simulink model "CCModel_61"  (R2024a)
settings: Solver=ode3  StartTime=0.0  StopTime=100  FixedStep=0.001  RelTol=1e-3  EnableMultiTasking=on
undefined symbols (not defined in the file or in its folder): DiscIntNeverNeededParam, Hecate_desVel1, Hecate_desVel2, Hecate_desVel3, Hecate_horShift, Hecate_period, Hecate_slope, Hecate_Transition1, Hecate_Transition2, Hecate_verShift, i, PME_qb, qb_map, RPM_qb, V
libraries: simulink x46
(part 4 of 11)

== system CCModel_61/Cruise Control/Version 5.0/Detect Change ==
  note: This subsystem detects either a change in the reference velocity, or the driver releasing one of the pedals. It outputs the time of the change, the value of u just before the change, and a boolean "hasChanged" value
  desired_velocity : Inport
  throttle_const : Inport  Port=2
  brake_const : Inport  Port=3
  Smoothed u : Inport  Port=4
  (False) : Constant  Value=0
  (True) : Constant
  AND : Logic  IconShape=distinctive  AllPortsSameDT=off  OutDataTypeStr=boolean
  Clock : Clock
  Delay : Delay  DelayLength=1
  Delay1 : Delay  DelayLength=1
  Detect Change : simulink/Logic and Bit Operations/Detect Change  vinit=0  OutDataTypeStr=boolean
  Detect Change1 : simulink/Logic and Bit Operations/Detect Change  vinit=0  OutDataTypeStr=boolean
  Max : MinMax  Function=max  Inputs=2
  OR : Logic  Operator=OR  IconShape=distinctive  AllPortsSameDT=off  OutDataTypeStr=boolean
  Pedal_threshold : Constant
  Scope : Scope
  Subtract : Sum  Inputs=+-
  Switch : Switch  Criteria=u2 > Threshold  SaturateOnIntegerOverflow=off  InputSameDT=off
  Switch1 : Switch  Criteria=u2 > Threshold  SaturateOnIntegerOverflow=off  InputSameDT=off
  Switch2 : Switch  Criteria=u2 > Threshold  SaturateOnIntegerOverflow=off  InputSameDT=off
  Change_time : Outport
  Old u : Outport  Port=2
  hasChanged : Outport  Port=3
  wires:
  desired_velocity/1 -> Detect Change/1
  Detect Change/1 -> OR/1
  OR/1 -> Switch/2, Switch2/2, hasChanged/1
  Switch1/1 -> Detect Change1/1, Delay1/1
  AND/1 -> OR/2
  Clock/1 -> Switch/1
  Max/1 -> Subtract/1
  (True)/1 -> Switch1/1
  brake_const/1 -> Max/2
  Pedal_threshold/1 -> Subtract/2
  Subtract/1 -> Switch1/2
  (False)/1 -> Switch1/3
  throttle_const/1 -> Max/1
  Switch2/1 -> Switch2/3, Old u/1
  Delay/1 -> Switch2/1
  Switch/1 -> Switch/3, Scope/1, Change_time/1
  Smoothed u/1 -> Delay/1
  Detect Change1/1 -> AND/2
  Delay1/1 -> AND/1

== system CCModel_61/Cruise Control/Version 5.0/PID Controller ==
  note: Typical PID controller, outputs a value between -100 and 100
  error : Inport
  Grade : Inport  Port=2
  Add : Sum
  Add1 : Sum
  Derivative : Derivative
  GKi : Gain  Gain=0
  GKp : Gain  Gain=3
  Integrator : Integrator
  Integrator1 : Integrator
  Kd : Gain  Gain=0.1
  Ki : Gain  Gain=0.03
  Kp : Gain  Gain=3
  Saturation : Saturate  UpperLimit=100  LowerLimit=-100
  Sum : Sum  Inputs=+++
  u : Outport
  wires:
  Integrator/1 -> Ki/1
  error/1 -> Integrator/1, Kp/1, Derivative/1  "D"
  Kp/1 -> Sum/2  "P"
  Ki/1 -> Sum/1  "I"
  Saturation/1 -> u/1
  Derivative/1 -> Kd/1
  Kd/1 -> Sum/3  "D"
  Sum/1 -> Add1/1
  Add1/1 -> Saturation/1
  Grade/1 -> Integrator1/1, GKp/1
  Integrator1/1 -> GKi/1
  GKi/1 -> Add/1
  GKp/1 -> Add/2
  Add/1 -> Add1/2

== system CCModel_61/Cruise Control/Version 5.0/Sigmoid ==
  note: This whole part is just to eliminate weird cancellation errors that were happening
  note: This system smooths out curves using the sigmoid equation shown above.
      | u1 is "Old u" which is the last value u had when change was detected.
      | u2 is "New u" which is the current output being given by the PID controller.
      | x is the time elapsed since the last change
      | k is the "sigmoid gain" which dictates how fast the transition occurs
  Change_time : Inport
  Old u : Inport  Port=2
  New u : Inport  Port=3
  Add : Sum
  Add1 : Sum
  Add2 : Sum
  Clock : Clock
  Constant : Constant
  Constant1 : Constant
  Constant2 : Constant
  Divide : Product  Inputs=/*
  Divide1 : Product  Inputs=**
  Divide2 : Product  Inputs=/*
  Divide3 : Product  Inputs=**
  Gain : Gain  Gain=1000
  Gain1 : Gain  Gain=0.001
  K : Constant  Value=1.5
  Power{,1..3} (4 alike) : Math  Operator=pow
  Reciprocal : Product  Inputs=/
  Reciprocal1 : Product  Inputs=/
  Round : Rounding  Operator=round
  Scope : Scope  NumInputPorts=3
  Subtract : Sum  Inputs=-+
  Sum : Sum  Inputs=|-+
  u_out : Outport
  wires:
  Power1/1 -> Scope/3, Add/1
  Add/1 -> Power/1
  Clock/1 -> Sum/2
  Constant/1 -> Add/2
  Sum/1 -> Gain/1  "Elapsed Time"
  Reciprocal/1 -> Power/2
  Power/1 -> Divide/1
  Divide/1 -> Divide1/1  "Sigmoid Function"
  Add1/1 -> Power2/1
  Power3/1 -> Add1/1
  K/1 -> Scope/2, Reciprocal/1, Power1/2, Reciprocal1/1, Power3/2
  Reciprocal1/1 -> Power2/2
  Power2/1 -> Divide2/1
  Constant1/1 -> Add1/2
  Change_time/1 -> Sum/1
  Constant2/1 -> Subtract/2
  Divide2/1 -> Subtract/1  "Sigmoid Function"
  Divide1/1 -> Add2/1
  Add2/1 -> u_out/1
  New u/1 -> Divide1/2
  Old u/1 -> Divide3/2
  Subtract/1 -> Divide3/1
  Divide3/1 -> Add2/2
  Gain1/1 -> Power1/1, Divide/2, Scope/1, Divide2/2, Power3/1
  Gain/1 -> Round/1
  Round/1 -> Gain1/1

== system CCModel_61/Cruise Control/Version 5.0/Switches ==
  note: This subsystem determines the source of input, either the cruise control or the driver
      | It also determines for a given u if the brake or throttle should be applied
      | Lastly, it smooths out the cruise control brakes and throttles to prevent jerk peaks
  note: Apply sigmoid curving to the throttle and brake
  note: If u is positive, throttle is applied
      | If u is negative, brake is applied
      | Max gains prevent large jerks from happening
  note: If throttle or brake are above 5 the driver takes control of the system
  throttle_const : Inport
  u : Inport  Port=2
  brake_const : Inport  Port=3
  hasChanged : Inport  Port=4
  Grade : Inport  Port=5
  (False) : Constant  Value=0
  (True) : Constant
  Brake_Switch : Switch  Criteria=u2 > Threshold  SaturateOnIntegerOverflow=off  InputSameDT=off
  Brake_Switch2 : Switch  Criteria=u2 > Threshold  SaturateOnIntegerOverflow=off  InputSameDT=off
  Clock : Clock
  Clock1 : Clock
  Constant : Constant
  Constant3 : Constant  Value=0
  Delay1 : Delay  DelayLength=1
  Delay3 : Delay  DelayLength=1
  Gain : Gain  Gain=1/150
  Gain1 : Gain  Gain=4
  Gain2 : Gain  Gain=-1
  Max : MinMax  Function=max  Inputs=2
  Max Brake : Gain  Gain=-0.5
  Max Throttle : Gain  Commented=through  Gain=0.8
  Pedal_threshold : Constant  Value=5
  Sigmoid_brake : Subsystem
  Sigmoid_throttle : Subsystem
  Sqrt : Sqrt
  Square : Math  Operator=square
  Subtract : Sum  Inputs=+-
  Switch : Switch  Criteria=u2 > Threshold  SaturateOnIntegerOverflow=off  InputSameDT=off
  Switch{1..4} (4 alike) : Switch  Criteria=u2 > Threshold  Threshold=0.04  SaturateOnIntegerOverflow=off  InputSameDT=off
  Switch5 : Switch  Criteria=u2 > Threshold  SaturateOnIntegerOverflow=off  InputSameDT=off
  Switch6 : Switch  Criteria=u2 > Threshold  Threshold=2.5  SaturateOnIntegerOverflow=off  InputSameDT=off
  Throttle_Switch : Switch  Criteria=u2 > Threshold  SaturateOnIntegerOverflow=off  InputSameDT=off
  Throttle_Switch2 : Switch  Criteria=u2 > Threshold  SaturateOnIntegerOverflow=off  InputSameDT=off
  Throttle : Outport
  Brake : Outport  Port=2
  Source : Outport  Port=3
  wires:
  throttle_const/1 -> Throttle_Switch2/1, Max/1
  brake_const/1 -> Max/2, Brake_Switch2/1
  Max/1 -> Subtract/1
  Pedal_threshold/1 -> Subtract/2
  Subtract/1 -> Switch/2
  (True)/1 -> Switch/1
  (False)/1 -> Switch/3
  Switch/1 -> Brake_Switch2/2, Throttle_Switch2/2, Source/1
  u/1 -> Throttle_Switch/2, Square/1, Brake_Switch/2, Max Brake/1, Gain2/1
  Constant3/1 -> Brake_Switch/1, Throttle_Switch/3
  Throttle_Switch2/1 -> Throttle/1
  Brake_Switch2/1 -> Brake/1
  Switch1/1 -> Switch1/3, Sigmoid_throttle/1(Change_time)  "Time"
  Switch2/1 -> Switch2/3, Sigmoid_throttle/2(Old thr)  "Old throttle"
  Throttle_Switch/1 -> Sigmoid_throttle/3(New thr)  "Throttle"
  Sigmoid_throttle/1(throttle_out) -> Delay1/1, Throttle_Switch2/3  "Smoothed throttle"
  Clock/1 -> Switch1/1
  hasChanged/1 -> Switch4/2, Switch3/2, Switch1/2, Switch2/2
  Delay1/1 -> Switch2/1
  Switch3/1 -> Switch3/3, Sigmoid_brake/1(Change_time)  "Time"
  Brake_Switch/1 -> Sigmoid_brake/3(New brake)  "Brake"
  Clock1/1 -> Switch3/1
  Switch4/1 -> Switch4/3, Sigmoid_brake/2(Old brake)  "Old brake"
  Delay3/1 -> Switch4/1
  Sigmoid_brake/1(brake_out) -> Delay3/1, Brake_Switch2/3  "Smoothed Brake"
  Square/1 -> Gain/1
  Sqrt/1 -> Gain1/1
  Gain2/1 -> Sqrt/1
  Gain/1 -> Throttle_Switch/1
  Grade/1 -> Switch5/2, Switch6/2
  Gain1/1 -> Switch5/3
  Max Brake/1 -> Switch6/3
  Switch6/1 -> Switch5/1
  Switch5/1 -> Brake_Switch/3
  Constant/1 -> Switch6/1

== system CCModel_61/Cruise Control/Version 6.0/Detect Change ==
  note: This subsystem detects either a change in the reference velocity, or the driver releasing one of the pedals. It outputs the time of the change, the value of u just before the change, and a boolean "hasChanged" value
  desired_velocity : Inport
  throttle_const : Inport  Port=2
  brake_const : Inport  Port=3
  Smoothed u : Inport  Port=4
  (False) : Constant  Value=0
  (True) : Constant
  AND : Logic  IconShape=distinctive  AllPortsSameDT=off  OutDataTypeStr=boolean
  Clock : Clock
  Delay : Delay  DelayLength=1
  Delay1 : Delay  DelayLength=1
  Detect Change : simulink/Logic and Bit Operations/Detect Change  vinit=0  OutDataTypeStr=boolean
  Detect Change1 : simulink/Logic and Bit Operations/Detect Change  vinit=0  OutDataTypeStr=boolean
  Max : MinMax  Function=max  Inputs=2
  OR : Logic  Operator=OR  IconShape=distinctive  AllPortsSameDT=off  OutDataTypeStr=boolean
  Pedal_threshold : Constant
  Scope : Scope
  Subtract : Sum  Inputs=+-
  Switch : Switch  Criteria=u2 > Threshold  SaturateOnIntegerOverflow=off  InputSameDT=off
  Switch1 : Switch  Criteria=u2 > Threshold  SaturateOnIntegerOverflow=off  InputSameDT=off
  Switch2 : Switch  Criteria=u2 > Threshold  SaturateOnIntegerOverflow=off  InputSameDT=off
  Change_time : Outport
  Old u : Outport  Port=2
  hasChanged : Outport  Port=3
  wires:
  desired_velocity/1 -> Detect Change/1
  Detect Change/1 -> OR/1
  OR/1 -> Switch/2, Switch2/2, hasChanged/1
  Switch1/1 -> Detect Change1/1, Delay1/1
  AND/1 -> OR/2
  Clock/1 -> Switch/1
  Max/1 -> Subtract/1
  (True)/1 -> Switch1/1
  brake_const/1 -> Max/2
  Pedal_threshold/1 -> Subtract/2
  Subtract/1 -> Switch1/2
  (False)/1 -> Switch1/3
  throttle_const/1 -> Max/1
  Switch2/1 -> Switch2/3, Old u/1
  Delay/1 -> Switch2/1
  Switch/1 -> Switch/3, Scope/1, Change_time/1
  Smoothed u/1 -> Delay/1
  Detect Change1/1 -> AND/2
  Delay1/1 -> AND/1

== system CCModel_61/Cruise Control/Version 6.0/PID Controller ==
  note: Typical PID controller, outputs a value between -100 and 100
  error : Inport
  Grade : Inport  Port=2
  Add : Sum
  Add1 : Sum
  Derivative : Derivative
  GKi : Gain  Gain=0
  GKp : Gain  Gain=0
  Integrator : Integrator
  Integrator1 : Integrator
  Kd : Gain  Gain=0.1
  Ki : Gain  Gain=0.03
  Kp : Gain  Gain=5
  Saturation : Saturate  UpperLimit=100  LowerLimit=-100
  Sum : Sum  Inputs=+++
  u : Outport
  wires:
  Integrator/1 -> Ki/1
  error/1 -> Integrator/1, Kp/1, Derivative/1  "D"
  Kp/1 -> Sum/2  "P"
  Ki/1 -> Sum/1  "I"
  Saturation/1 -> u/1
  Derivative/1 -> Kd/1
  Kd/1 -> Sum/3  "D"
  Sum/1 -> Add1/1
  Add1/1 -> Saturation/1
  Grade/1 -> Integrator1/1, GKp/1
  Integrator1/1 -> GKi/1
  GKi/1 -> Add/1
  GKp/1 -> Add/2
  Add/1 -> Add1/2

== system CCModel_61/Cruise Control/Version 6.0/Sigmoid ==
  note: This whole part is just to eliminate weird cancellation errors that were happening
  note: This system smooths out curves using the sigmoid equation shown above.
      | u1 is "Old u" which is the last value u had when change was detected.
      | u2 is "New u" which is the current output being given by the PID controller.
      | x is the time elapsed since the last change
      | k is the "sigmoid gain" which dictates how fast the transition occurs
  Change_time : Inport
  Old u : Inport  Port=2
  New u : Inport  Port=3
  Add : Sum
  Add1 : Sum
  Add2 : Sum
  Clock : Clock
  Constant : Constant
  Constant1 : Constant
  Constant2 : Constant
  Divide : Product  Inputs=/*
  Divide1 : Product  Inputs=**
  Divide2 : Product  Inputs=/*
  Divide3 : Product  Inputs=**
  Gain : Gain  Gain=1000
  Gain1 : Gain  Gain=0.001
  K : Constant  Value=1.5
  Power{,1..3} (4 alike) : Math  Operator=pow
  Reciprocal : Product  Inputs=/
  Reciprocal1 : Product  Inputs=/
  Round : Rounding  Operator=round
  Scope : Scope  NumInputPorts=3
  Subtract : Sum  Inputs=-+
  Sum : Sum  Inputs=|-+
  u_out : Outport
  wires:
  Power1/1 -> Scope/3, Add/1
  Add/1 -> Power/1
  Clock/1 -> Sum/2
  Constant/1 -> Add/2
  Sum/1 -> Gain/1  "Elapsed Time"
  Reciprocal/1 -> Power/2
  Power/1 -> Divide/1
  Divide/1 -> Divide1/1  "Sigmoid Function"
  Add1/1 -> Power2/1
  Power3/1 -> Add1/1
  K/1 -> Scope/2, Reciprocal/1, Power1/2, Reciprocal1/1, Power3/2
  Reciprocal1/1 -> Power2/2
  Power2/1 -> Divide2/1
  Constant1/1 -> Add1/2
  Change_time/1 -> Sum/1
  Constant2/1 -> Subtract/2
  Divide2/1 -> Subtract/1  "Sigmoid Function"
  Divide1/1 -> Add2/1
  Add2/1 -> u_out/1
  New u/1 -> Divide1/2
  Old u/1 -> Divide3/2
  Subtract/1 -> Divide3/1
  Divide3/1 -> Add2/2
  Gain1/1 -> Power1/1, Divide/2, Scope/1, Divide2/2, Power3/1
  Gain/1 -> Round/1
  Round/1 -> Gain1/1

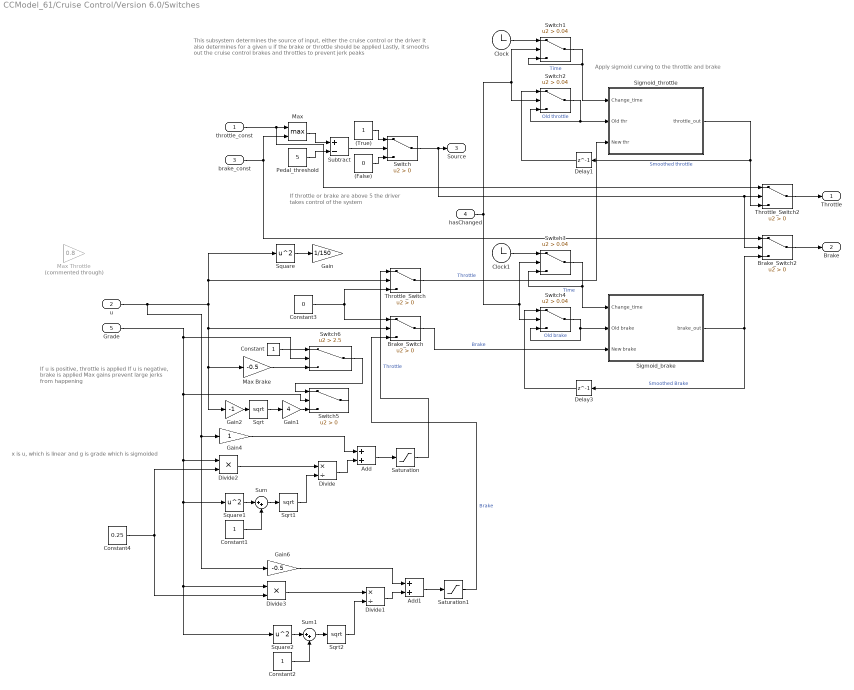
== system CCModel_61/Cruise Control/Version 6.0/Switches ==
  note: x is u, which is linear and g is grade which is sigmoided
  note: This subsystem determines the source of input, either the cruise control or the driver
      | It also determines for a given u if the brake or throttle should be applied
      | Lastly, it smooths out the cruise control brakes and throttles to prevent jerk peaks
  note: Apply sigmoid curving to the throttle and brake
  note: If u is positive, throttle is applied
      | If u is negative, brake is applied
      | Max gains prevent large jerks from happening
  note: If throttle or brake are above 5 the driver takes control of the system
  throttle_const : Inport
  u : Inport  Port=2
  brake_const : Inport  Port=3
  hasChanged : Inport  Port=4
  Grade : Inport  Port=5
  (False) : Constant  Value=0
  (True) : Constant
  Add : Sum
  Add1 : Sum
  Brake_Switch : Switch  Criteria=u2 > Threshold  SaturateOnIntegerOverflow=off  InputSameDT=off
  Brake_Switch2 : Switch  Criteria=u2 > Threshold  SaturateOnIntegerOverflow=off  InputSameDT=off
  Clock : Clock
  Clock1 : Clock
  Constant : Constant
  Constant1 : Constant
  Constant2 : Constant
  Constant3 : Constant  Value=0
  Constant4 : Constant  Value=0.25
  Delay1 : Delay  DelayLength=1
  Delay3 : Delay  DelayLength=1
  Divide : Product  Inputs=*/
  Divide1 : Product  Inputs=*/
  Divide2 : Product  Inputs=**
  Divide3 : Product  Inputs=**
  Gain : Gain  Gain=1/150
  Gain1 : Gain  Gain=4
  Gain2 : Gain  Gain=-1
  Gain4 : Gain
  Gain6 : Gain  Gain=-0.5
  Max : MinMax  Function=max  Inputs=2
  Max Brake : Gain  Gain=-0.5
  Max Throttle : Gain  Commented=through  Gain=0.8
  Pedal_threshold : Constant  Value=5
  Saturation : Saturate  UpperLimit=100  LowerLimit=0
  Saturation1 : Saturate  UpperLimit=100  LowerLimit=0
  Sigmoid_brake : Subsystem
  Sigmoid_throttle : Subsystem
  Sqrt : Sqrt
  Sqrt1 : Sqrt
  Sqrt2 : Sqrt
  Square : Math  Operator=square
  Square1 : Math  Operator=square
  Square2 : Math  Operator=square
  Subtract : Sum  Inputs=+-
  Sum : Sum  Inputs=|++
  Sum1 : Sum  Inputs=|++
  Switch : Switch  Criteria=u2 > Threshold  SaturateOnIntegerOverflow=off  InputSameDT=off
  Switch{1..4} (4 alike) : Switch  Criteria=u2 > Threshold  Threshold=0.04  SaturateOnIntegerOverflow=off  InputSameDT=off
  Switch5 : Switch  Criteria=u2 > Threshold  SaturateOnIntegerOverflow=off  InputSameDT=off
  Switch6 : Switch  Criteria=u2 > Threshold  Threshold=2.5  SaturateOnIntegerOverflow=off  InputSameDT=off
  Throttle_Switch : Switch  Criteria=u2 > Threshold  SaturateOnIntegerOverflow=off  InputSameDT=off
  Throttle_Switch2 : Switch  Criteria=u2 > Threshold  SaturateOnIntegerOverflow=off  InputSameDT=off
  Throttle : Outport
  Brake : Outport  Port=2
  Source : Outport  Port=3
  wires:
  throttle_const/1 -> Throttle_Switch2/1, Max/1
  brake_const/1 -> Max/2, Brake_Switch2/1
  Max/1 -> Subtract/1
  Pedal_threshold/1 -> Subtract/2
  Subtract/1 -> Switch/2
  (True)/1 -> Switch/1
  (False)/1 -> Switch/3
  Switch/1 -> Brake_Switch2/2, Throttle_Switch2/2, Source/1
  u/1 -> Gain6/1, Gain4/1, Throttle_Switch/2, Square/1, Brake_Switch/2, Max Brake/1, Gain2/1
  Constant3/1 -> Brake_Switch/1, Throttle_Switch/3
  Throttle_Switch2/1 -> Throttle/1
  Brake_Switch2/1 -> Brake/1
  Switch1/1 -> Switch1/3, Sigmoid_throttle/1(Change_time)  "Time"
  Switch2/1 -> Switch2/3, Sigmoid_throttle/2(Old thr)  "Old throttle"
  Throttle_Switch/1 -> Sigmoid_throttle/3(New thr)  "Throttle"
  Sigmoid_throttle/1(throttle_out) -> Delay1/1, Throttle_Switch2/3  "Smoothed throttle"
  Clock/1 -> Switch1/1
  hasChanged/1 -> Switch4/2, Switch3/2, Switch1/2, Switch2/2
  Delay1/1 -> Switch2/1
  Switch3/1 -> Switch3/3, Sigmoid_brake/1(Change_time)  "Time"
  Brake_Switch/1 -> Sigmoid_brake/3(New brake)  "Brake"
  Clock1/1 -> Switch3/1
  Switch4/1 -> Switch4/3, Sigmoid_brake/2(Old brake)  "Old brake"
  Delay3/1 -> Switch4/1
  Sigmoid_brake/1(brake_out) -> Delay3/1, Brake_Switch2/3  "Smoothed Brake"
  Square/1 -> Gain/1
  Sqrt/1 -> Gain1/1
  Gain2/1 -> Sqrt/1
  Gain1/1 -> Switch5/3
  Max Brake/1 -> Switch6/3
  Switch6/1 -> Switch5/1
  Constant/1 -> Switch6/1
  Square1/1 -> Sum/1
  Constant1/1 -> Sum/2
  Sum/1 -> Sqrt1/1
  Divide2/1 -> Divide/1
  Sqrt1/1 -> Divide/2
  Gain4/1 -> Add/1
  Divide/1 -> Add/2
  Add/1 -> Saturation/1
  Saturation/1 -> Throttle_Switch/1  "Throttle"
  Square2/1 -> Sum1/1
  Gain6/1 -> Add1/1
  Divide1/1 -> Add1/2
  Constant2/1 -> Sum1/2
  Divide3/1 -> Divide1/1
  Sum1/1 -> Sqrt2/1
  Add1/1 -> Saturation1/1
  Sqrt2/1 -> Divide1/2
  Grade/1 -> Switch5/2, Divide2/1, Square1/1, Divide3/1, Square2/1, Switch6/2
  Saturation1/1 -> Brake_Switch/3  "Brake"
  Constant4/1 -> Divide3/2, Divide2/2

== system CCModel_61/Cruise Control/Version 6.1/Detect Change ==
  note: This subsystem detects either a change in the reference velocity, or the driver releasing one of the pedals. It outputs the time of the change, the value of u just before the change, and a boolean "hasChanged" value
  desired_velocity : Inport
  throttle_const : Inport  Port=2
  brake_const : Inport  Port=3
  Smoothed u : Inport  Port=4
  (False) : Constant  Value=0
  (True) : Constant
  AND : Logic  IconShape=distinctive  AllPortsSameDT=off  OutDataTypeStr=boolean
  Clock : Clock
  Delay : Delay  DelayLength=1
  Delay1 : Delay  DelayLength=1
  Detect Change : simulink/Logic and Bit Operations/Detect Change  vinit=0  OutDataTypeStr=boolean
  Detect Change1 : simulink/Logic and Bit Operations/Detect Change  vinit=0  OutDataTypeStr=boolean
  Max : MinMax  Function=max  Inputs=2
  OR : Logic  Operator=OR  IconShape=distinctive  AllPortsSameDT=off  OutDataTypeStr=boolean
  Pedal_threshold : Constant
  Scope : Scope
  Subtract : Sum  Inputs=+-
  Switch : Switch  Criteria=u2 > Threshold  SaturateOnIntegerOverflow=off  InputSameDT=off
  Switch1 : Switch  Criteria=u2 > Threshold  SaturateOnIntegerOverflow=off  InputSameDT=off
  Switch2 : Switch  Criteria=u2 > Threshold  SaturateOnIntegerOverflow=off  InputSameDT=off
  Change_time : Outport
  Old u : Outport  Port=2
  hasChanged : Outport  Port=3
  wires:
  desired_velocity/1 -> Detect Change/1
  Detect Change/1 -> OR/1
  OR/1 -> Switch/2, Switch2/2, hasChanged/1
  Switch1/1 -> Detect Change1/1, Delay1/1
  AND/1 -> OR/2
  Clock/1 -> Switch/1
  Max/1 -> Subtract/1
  (True)/1 -> Switch1/1
  brake_const/1 -> Max/2
  Pedal_threshold/1 -> Subtract/2
  Subtract/1 -> Switch1/2
  (False)/1 -> Switch1/3
  throttle_const/1 -> Max/1
  Switch2/1 -> Switch2/3, Old u/1
  Delay/1 -> Switch2/1
  Switch/1 -> Switch/3, Scope/1, Change_time/1
  Smoothed u/1 -> Delay/1
  Detect Change1/1 -> AND/2
  Delay1/1 -> AND/1

== system CCModel_61/Cruise Control/Version 6.1/PID Controller ==
  note: Typical PID controller, outputs a value between -100 and 100
  error : Inport
  Grade : Inport  Port=2
  Add : Sum
  Add1 : Sum
  Derivative : Derivative
  GKi : Gain  Gain=0
  GKp : Gain  Gain=0
  Integrator : Integrator
  Integrator1 : Integrator
  Kd : Gain  Gain=0.1
  Ki : Gain  Gain=0.03
  Kp : Gain  Gain=3
  Saturation : Saturate  UpperLimit=100  LowerLimit=-100
  Scope : Scope  NumInputPorts=2
  Scope1 : Scope  NumInputPorts=3
  Sum : Sum  Inputs=+++
  u : Outport
  P : Outport  Port=2
  wires:
  Integrator/1 -> Ki/1
  error/1 -> Scope/1, Integrator/1, Kp/1, Derivative/1  "D"
  Kp/1 -> P/1, Scope1/1, Sum/2  "P"
  Ki/1 -> Sum/1, Scope1/2  "I"
  Saturation/1 -> u/1
  Derivative/1 -> Kd/1
  Kd/1 -> Scope1/3, Sum/3  "D"
  Sum/1 -> Add1/1, Scope/2
  Add1/1 -> Saturation/1
  Grade/1 -> Integrator1/1, GKp/1
  Integrator1/1 -> GKi/1
  GKi/1 -> Add/1
  GKp/1 -> Add/2
  Add/1 -> Add1/2

== system CCModel_61/Cruise Control/Version 6.1/Sigmoid ==
  note: This whole part is just to eliminate weird cancellation errors that were happening
  note: This system smooths out curves using the sigmoid equation shown above.
      | u1 is "Old u" which is the last value u had when change was detected.
      | u2 is "New u" which is the current output being given by the PID controller.
      | x is the time elapsed since the last change
      | k is the "sigmoid gain" which dictates how fast the transition occurs
  Change_time : Inport
  Old u : Inport  Port=2
  New u : Inport  Port=3
  Add : Sum
  Add1 : Sum
  Add2 : Sum
  Clock : Clock
  Constant : Constant
  Constant1 : Constant
  Constant2 : Constant
  Divide : Product  Inputs=/*
  Divide1 : Product  Inputs=**
  Divide2 : Product  Inputs=/*
  Divide3 : Product  Inputs=**
  Gain : Gain  Gain=1000
  Gain1 : Gain  Gain=0.001
  K : Constant  Value=1.5
  Power{,1..3} (4 alike) : Math  Operator=pow
  Reciprocal : Product  Inputs=/
  Reciprocal1 : Product  Inputs=/
  Round : Rounding  Operator=round
  Scope : Scope  NumInputPorts=3
  Subtract : Sum  Inputs=-+
  Sum : Sum  Inputs=|-+
  u_out : Outport
  wires:
  Power1/1 -> Scope/3, Add/1
  Add/1 -> Power/1
  Clock/1 -> Sum/2
  Constant/1 -> Add/2
  Sum/1 -> Gain/1  "Elapsed Time"
  Reciprocal/1 -> Power/2
  Power/1 -> Divide/1
  Divide/1 -> Divide1/1  "Sigmoid Function"
  Add1/1 -> Power2/1
  Power3/1 -> Add1/1
  K/1 -> Scope/2, Reciprocal/1, Power1/2, Reciprocal1/1, Power3/2
  Reciprocal1/1 -> Power2/2
  Power2/1 -> Divide2/1
  Constant1/1 -> Add1/2
  Change_time/1 -> Sum/1
  Constant2/1 -> Subtract/2
  Divide2/1 -> Subtract/1  "Sigmoid Function"
  Divide1/1 -> Add2/1
  Add2/1 -> u_out/1
  New u/1 -> Divide1/2
  Old u/1 -> Divide3/2
  Subtract/1 -> Divide3/1
  Divide3/1 -> Add2/2
  Gain1/1 -> Power1/1, Divide/2, Scope/1, Divide2/2, Power3/1
  Gain/1 -> Round/1
  Round/1 -> Gain1/1

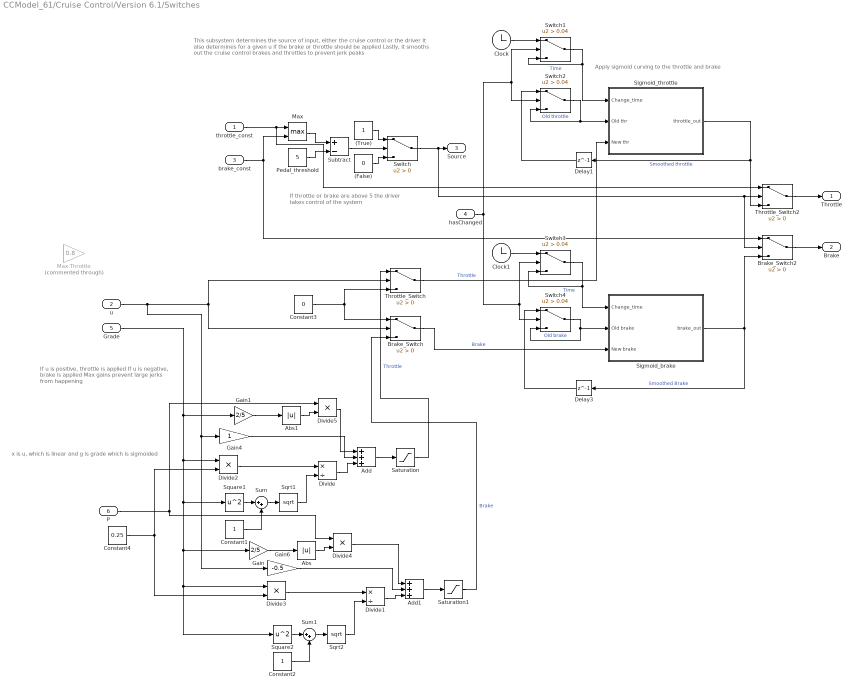
== system CCModel_61/Cruise Control/Version 6.1/Switches ==
  note: x is u, which is linear and g is grade which is sigmoided
  note: This subsystem determines the source of input, either the cruise control or the driver
      | It also determines for a given u if the brake or throttle should be applied
      | Lastly, it smooths out the cruise control brakes and throttles to prevent jerk peaks
  note: Apply sigmoid curving to the throttle and brake
  note: If u is positive, throttle is applied
      | If u is negative, brake is applied
      | Max gains prevent large jerks from happening
  note: If throttle or brake are above 5 the driver takes control of the system
  throttle_const : Inport
  u : Inport  Port=2
  brake_const : Inport  Port=3
  hasChanged : Inport  Port=4
  Grade : Inport  Port=5
  P : Inport  Port=6
  (False) : Constant  Value=0
  (True) : Constant
  Abs : Abs  SaturateOnIntegerOverflow=off
  Abs1 : Abs  SaturateOnIntegerOverflow=off
  Add : Sum  Inputs=+++
  Add1 : Sum  Inputs=+++
  Brake_Switch : Switch  Criteria=u2 > Threshold  SaturateOnIntegerOverflow=off  InputSameDT=off
  Brake_Switch2 : Switch  Criteria=u2 > Threshold  SaturateOnIntegerOverflow=off  InputSameDT=off
  Clock : Clock
  Clock1 : Clock
  Constant1 : Constant
  Constant2 : Constant
  Constant3 : Constant  Value=0
  Constant4 : Constant  Value=0.25
  Delay1 : Delay  DelayLength=1
  Delay3 : Delay  DelayLength=1
  Divide : Product  Inputs=*/
  Divide1 : Product  Inputs=*/
  Divide{2..5} (4 alike) : Product  Inputs=**
  Gain : Gain  Gain=2/5
  Gain1 : Gain  Gain=2/5
  Gain4 : Gain
  Gain6 : Gain  Gain=-0.5
  Max : MinMax  Function=max  Inputs=2
  Max Throttle : Gain  Commented=through  Gain=0.8
  Pedal_threshold : Constant  Value=5
  Saturation : Saturate  UpperLimit=100  LowerLimit=0
  Saturation1 : Saturate  UpperLimit=100  LowerLimit=0
  Sigmoid_brake : Subsystem
  Sigmoid_throttle : Subsystem
  Sqrt1 : Sqrt
  Sqrt2 : Sqrt
  Square1 : Math  Operator=square
  Square2 : Math  Operator=square
  Subtract : Sum  Inputs=+-
  Sum : Sum  Inputs=|++
  Sum1 : Sum  Inputs=|++
  Switch : Switch  Criteria=u2 > Threshold  SaturateOnIntegerOverflow=off  InputSameDT=off
  Switch{1..4} (4 alike) : Switch  Criteria=u2 > Threshold  Threshold=0.04  SaturateOnIntegerOverflow=off  InputSameDT=off
  Throttle_Switch : Switch  Criteria=u2 > Threshold  SaturateOnIntegerOverflow=off  InputSameDT=off
  Throttle_Switch2 : Switch  Criteria=u2 > Threshold  SaturateOnIntegerOverflow=off  InputSameDT=off
  Throttle : Outport
  Brake : Outport  Port=2
  Source : Outport  Port=3
  wires:
  throttle_const/1 -> Throttle_Switch2/1, Max/1
  brake_const/1 -> Max/2, Brake_Switch2/1
  Max/1 -> Subtract/1
  Pedal_threshold/1 -> Subtract/2
  Subtract/1 -> Switch/2
  (True)/1 -> Switch/1
  (False)/1 -> Switch/3
  Switch/1 -> Brake_Switch2/2, Throttle_Switch2/2, Source/1
  u/1 -> Gain6/1, Gain4/1, Throttle_Switch/2, Brake_Switch/2
  Constant3/1 -> Brake_Switch/1, Throttle_Switch/3
  Throttle_Switch2/1 -> Throttle/1
  Brake_Switch2/1 -> Brake/1
  Switch1/1 -> Switch1/3, Sigmoid_throttle/1(Change_time)  "Time"
  Switch2/1 -> Switch2/3, Sigmoid_throttle/2(Old thr)  "Old throttle"
  Throttle_Switch/1 -> Sigmoid_throttle/3(New thr)  "Throttle"
  Sigmoid_throttle/1(throttle_out) -> Delay1/1, Throttle_Switch2/3  "Smoothed throttle"
  Clock/1 -> Switch1/1
  hasChanged/1 -> Switch4/2, Switch3/2, Switch1/2, Switch2/2
  Delay1/1 -> Switch2/1
  Switch3/1 -> Switch3/3, Sigmoid_brake/1(Change_time)  "Time"
  Brake_Switch/1 -> Sigmoid_brake/3(New brake)  "Brake"
  Clock1/1 -> Switch3/1
  Switch4/1 -> Switch4/3, Sigmoid_brake/2(Old brake)  "Old brake"
  Delay3/1 -> Switch4/1
  Sigmoid_brake/1(brake_out) -> Delay3/1, Brake_Switch2/3  "Smoothed Brake"
  Square1/1 -> Sum/1
  Constant1/1 -> Sum/2
  Sum/1 -> Sqrt1/1
  Divide2/1 -> Divide/1
  Sqrt1/1 -> Divide/2
  Gain4/1 -> Add/2
  Divide/1 -> Add/3
  Add/1 -> Saturation/1
  Saturation/1 -> Throttle_Switch/1  "Throttle"
  Square2/1 -> Sum1/1
  Gain6/1 -> Add1/2
  Divide1/1 -> Add1/3
  Constant2/1 -> Sum1/2
  Divide3/1 -> Divide1/1
  Sum1/1 -> Sqrt2/1
  Add1/1 -> Saturation1/1
  Sqrt2/1 -> Divide1/2
  Grade/1 -> Gain1/1, Divide2/1, Square1/1, Gain/1, Divide3/1, Square2/1
  Saturation1/1 -> Brake_Switch/3  "Brake"
  Constant4/1 -> Divide3/2, Divide2/2
  Divide4/1 -> Add1/1
  Gain/1 -> Abs/1
  Abs/1 -> Divide4/2
  Abs1/1 -> Divide5/2
  Gain1/1 -> Abs1/1
  Divide5/1 -> Add/1
  P/1 -> Divide4/1, Divide5/1

== system CCModel_61/Cruise Control/Version 6.2/Detect Change ==
  note: This subsystem detects either a change in the reference velocity, or the driver releasing one of the pedals. It outputs the time of the change, the value of u just before the change, and a boolean "hasChanged" value
  desired_velocity : Inport
  throttle_const : Inport  Port=2
  brake_const : Inport  Port=3
  Smoothed u : Inport  Port=4
  (False) : Constant  Value=0
  (True) : Constant
  AND : Logic  IconShape=distinctive  AllPortsSameDT=off  OutDataTypeStr=boolean
  Clock : Clock
  Delay{,1..3} (4 alike) : Delay  DelayLength=1
  Detect Change : simulink/Logic and Bit Operations/Detect Change  vinit=0  OutDataTypeStr=boolean
  Detect Change1 : simulink/Logic and Bit Operations/Detect Change  vinit=0  OutDataTypeStr=boolean
  Max : MinMax  Function=max  Inputs=2
  OR : Logic  Operator=OR  IconShape=distinctive  AllPortsSameDT=off  OutDataTypeStr=boolean
  Pedal_threshold : Constant
  Scope : Scope
  Subtract : Sum  Inputs=+-
  Switch : Switch  Criteria=u2 > Threshold  SaturateOnIntegerOverflow=off  InputSameDT=off
  Switch1 : Switch  Criteria=u2 > Threshold  SaturateOnIntegerOverflow=off  InputSameDT=off
  Switch2 : Switch  Criteria=u2 > Threshold  SaturateOnIntegerOverflow=off  InputSameDT=off
  Change_time : Outport
  Old u : Outport  Port=2
  hasChanged : Outport  Port=3
  wires:
  desired_velocity/1 -> Detect Change/1
  Detect Change/1 -> OR/1
  OR/1 -> Switch/2, Switch2/2, hasChanged/1
  Switch1/1 -> Detect Change1/1, Delay1/1
  AND/1 -> OR/2
  Clock/1 -> Switch/1
  Max/1 -> Subtract/1
  (True)/1 -> Switch1/1
  brake_const/1 -> Max/2
  Pedal_threshold/1 -> Subtract/2
  Subtract/1 -> Switch1/2
  (False)/1 -> Switch1/3
  throttle_const/1 -> Max/1
  Switch2/1 -> Delay3/1, Old u/1
  Delay/1 -> Switch2/1
  Switch/1 -> Delay2/1, Scope/1, Change_time/1
  Smoothed u/1 -> Delay/1
  Detect Change1/1 -> AND/2
  Delay1/1 -> AND/1
  Delay2/1 -> Switch/3
  Delay3/1 -> Switch2/3

== system CCModel_61/Cruise Control/Version 6.2/PID Controller ==
  note: Typical PID controller, outputs a value between -100 and 100
  error : Inport
  Grade : Inport  Port=2
  Add : Sum
  Add1 : Sum
  Derivative : Derivative
  GKi : Gain  Gain=0
  GKp : Gain  Gain=0
  Integrator : Integrator
  Integrator1 : Integrator
  Kd : Gain  Gain=0.1
  Ki : Gain  Gain=0.03
  Kp : Gain  Gain=3
  Saturation : Saturate  UpperLimit=100  LowerLimit=-100
  Scope : Scope  NumInputPorts=2
  Scope1 : Scope  NumInputPorts=3
  Sum : Sum  Inputs=+++
  u : Outport
  P : Outport  Port=2
  wires:
  Integrator/1 -> Ki/1
  error/1 -> Scope/1, Integrator/1, Kp/1, Derivative/1  "D"
  Kp/1 -> P/1, Scope1/1, Sum/2  "P"
  Ki/1 -> Sum/1, Scope1/2  "I"
  Saturation/1 -> u/1
  Derivative/1 -> Kd/1
  Kd/1 -> Scope1/3, Sum/3  "D"
  Sum/1 -> Add1/1, Scope/2
  Add1/1 -> Saturation/1
  Grade/1 -> Integrator1/1, GKp/1
  Integrator1/1 -> GKi/1
  GKi/1 -> Add/1
  GKp/1 -> Add/2
  Add/1 -> Add1/2

== system CCModel_61/Cruise Control/Version 6.2/Sigmoid ==
  note: This whole part is just to eliminate weird cancellation errors that were happening
  note: This system smooths out curves using the sigmoid equation shown above.
      | u1 is "Old u" which is the last value u had when change was detected.
      | u2 is "New u" which is the current output being given by the PID controller.
      | x is the time elapsed since the last change
      | k is the "sigmoid gain" which dictates how fast the transition occurs
  Change_time : Inport
  Old u : Inport  Port=2
  New u : Inport  Port=3
  Add : Sum
  Add1 : Sum
  Add2 : Sum
  Clock : Clock
  Constant : Constant
  Constant1 : Constant
  Constant2 : Constant
  Divide : Product  Inputs=/*
  Divide1 : Product  Inputs=**
  Divide2 : Product  Inputs=/*
  Divide3 : Product  Inputs=**
  Gain : Gain  Gain=1000
  Gain1 : Gain  Gain=0.001
  K : Constant  Value=1.5
  Power{,1..3} (4 alike) : Math  Operator=pow
  Reciprocal : Product  Inputs=/
  Reciprocal1 : Product  Inputs=/
  Round : Rounding  Operator=round
  Scope : Scope  NumInputPorts=3
  Subtract : Sum  Inputs=-+
  Sum : Sum  Inputs=|-+
  u_out : Outport
  wires:
  Power1/1 -> Scope/3, Add/1
  Add/1 -> Power/1
  Clock/1 -> Sum/2
  Constant/1 -> Add/2
  Sum/1 -> Gain/1  "Elapsed Time"
  Reciprocal/1 -> Power/2
  Power/1 -> Divide/1
  Divide/1 -> Divide1/1  "Sigmoid Function"
  Add1/1 -> Power2/1
  Power3/1 -> Add1/1
  K/1 -> Scope/2, Reciprocal/1, Power1/2, Reciprocal1/1, Power3/2
  Reciprocal1/1 -> Power2/2
  Power2/1 -> Divide2/1
  Constant1/1 -> Add1/2
  Change_time/1 -> Sum/1
  Constant2/1 -> Subtract/2
  Divide2/1 -> Subtract/1  "Sigmoid Function"
  Divide1/1 -> Add2/1
  Add2/1 -> u_out/1
  New u/1 -> Divide1/2
  Old u/1 -> Divide3/2
  Subtract/1 -> Divide3/1
  Divide3/1 -> Add2/2
  Gain1/1 -> Power1/1, Divide/2, Scope/1, Divide2/2, Power3/1
  Gain/1 -> Round/1
  Round/1 -> Gain1/1

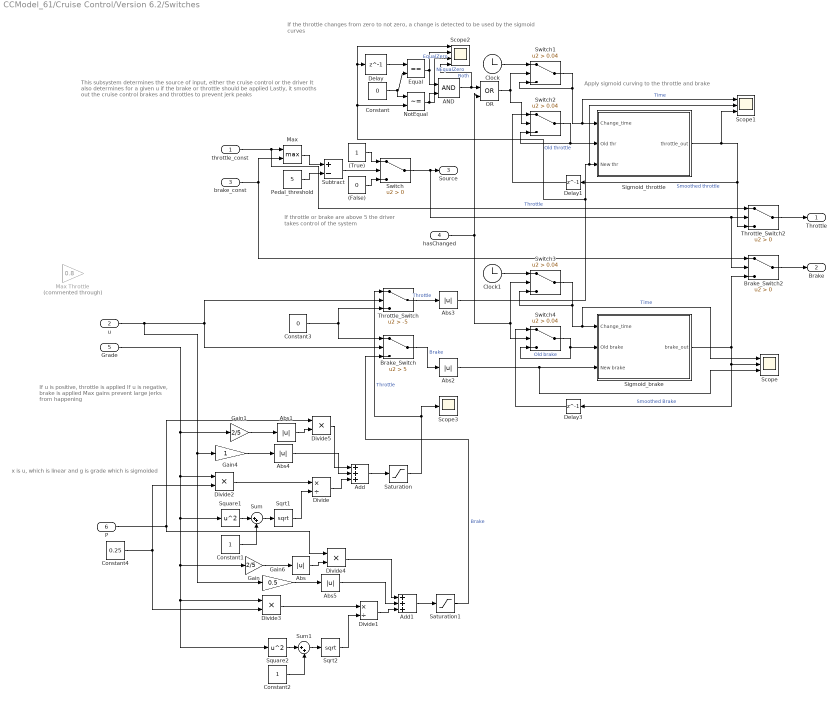
== system CCModel_61/Cruise Control/Version 6.2/Switches ==
  note: If the throttle changes from zero to not zero, a change is detected to be used by the sigmoid curves
  note: x is u, which is linear and g is grade which is sigmoided
  note: This subsystem determines the source of input, either the cruise control or the driver
      | It also determines for a given u if the brake or throttle should be applied
      | Lastly, it smooths out the cruise control brakes and throttles to prevent jerk peaks
  note: Apply sigmoid curving to the throttle and brake
  note: If u is positive, throttle is applied
      | If u is negative, brake is applied
      | Max gains prevent large jerks from happening
  note: If throttle or brake are above 5 the driver takes control of the system
  throttle_const : Inport
  u : Inport  Port=2
  brake_const : Inport  Port=3
  hasChanged : Inport  Port=4
  Grade : Inport  Port=5
  P : Inport  Port=6
  (False) : Constant  Value=0
  (True) : Constant
  AND : Logic  IconShape=distinctive  AllPortsSameDT=off  OutDataTypeStr=boolean
  Abs{,1..5} (6 alike) : Abs  SaturateOnIntegerOverflow=off
  Add : Sum  Inputs=+++
  Add1 : Sum  Inputs=+++
  Brake_Switch : Switch  Criteria=u2 > Threshold  Threshold=5  SaturateOnIntegerOverflow=off  InputSameDT=off
  Brake_Switch2 : Switch  Criteria=u2 > Threshold  SaturateOnIntegerOverflow=off  InputSameDT=off
  Clock : Clock
  Clock1 : Clock
  Constant : Constant  Value=0
  Constant1 : Constant
  Constant2 : Constant
  Constant3 : Constant  Value=0
  Constant4 : Constant  Value=0.25
  Delay : Delay  DelayLength=1
  Delay1 : Delay  DelayLength=1
  Delay3 : Delay  DelayLength=1
  Divide : Product  Inputs=*/
  Divide1 : Product  Inputs=*/
  Divide{2..5} (4 alike) : Product  Inputs=**
  Equal : RelationalOperator  Operator===  OutDataTypeStr=boolean  RndMeth=Simplest  InputSameDT=off
  Gain : Gain  Gain=2/5
  Gain1 : Gain  Gain=2/5
  Gain4 : Gain
  Gain6 : Gain  Gain=0.5
  Max : MinMax  Function=max  Inputs=2
  Max Throttle : Gain  Commented=through  Gain=0.8
  NotEqual : RelationalOperator  Operator=~=  OutDataTypeStr=boolean  RndMeth=Simplest  InputSameDT=off
  OR : Logic  Operator=OR  IconShape=distinctive  AllPortsSameDT=off  OutDataTypeStr=boolean
  Pedal_threshold : Constant  Value=5
  Saturation : Saturate  UpperLimit=100  LowerLimit=0
  Saturation1 : Saturate  UpperLimit=100  LowerLimit=0
  Scope : Scope  NumInputPorts=3
  Scope1 : Scope  NumInputPorts=3
  Scope2 : Scope  NumInputPorts=4
  Scope3 : Scope
  Sigmoid_brake : Subsystem
  Sigmoid_throttle : Subsystem
  Sqrt1 : Sqrt
  Sqrt2 : Sqrt
  Square1 : Math  Operator=square
  Square2 : Math  Operator=square
  Subtract : Sum  Inputs=+-
  Sum : Sum  Inputs=|++
  Sum1 : Sum  Inputs=|++
  Switch : Switch  Criteria=u2 > Threshold  SaturateOnIntegerOverflow=off  InputSameDT=off
  Switch{1..4} (4 alike) : Switch  Criteria=u2 > Threshold  Threshold=0.04  SaturateOnIntegerOverflow=off  InputSameDT=off
  Throttle_Switch : Switch  Criteria=u2 > Threshold  Threshold=-5  SaturateOnIntegerOverflow=off  InputSameDT=off
  Throttle_Switch2 : Switch  Criteria=u2 > Threshold  SaturateOnIntegerOverflow=off  InputSameDT=off
  Throttle : Outport
  Brake : Outport  Port=2
  Source : Outport  Port=3
  wires:
  throttle_const/1 -> Throttle_Switch2/1, Max/1  "Throttle"
  brake_const/1 -> Max/2, Brake_Switch2/1
  Max/1 -> Subtract/1
  Pedal_threshold/1 -> Subtract/2
  Subtract/1 -> Switch/2
  (True)/1 -> Switch/1
  (False)/1 -> Switch/3
  Switch/1 -> Brake_Switch2/2, Throttle_Switch2/2, Source/1
  u/1 -> Gain6/1, Gain4/1, Throttle_Switch/2, Brake_Switch/2
  Constant3/1 -> Brake_Switch/1, Throttle_Switch/3
  Throttle_Switch2/1 -> Throttle/1
  Brake_Switch2/1 -> Brake/1
  Switch1/1 -> Switch1/3, Scope1/1, Sigmoid_throttle/1(Change_time)  "Time"
  Switch2/1 -> Switch2/3, Sigmoid_throttle/2(Old thr)  "Old throttle"
  Throttle_Switch/1 -> Abs3/1  "Throttle"
  Sigmoid_throttle/1(throttle_out) -> Scope1/3, Delay1/1, Throttle_Switch2/3  "Smoothed throttle"
  Clock/1 -> Switch1/1
  hasChanged/1 -> OR/2, Switch4/2, Switch3/2
  Delay1/1 -> Switch2/1
  Switch3/1 -> Switch3/3, Scope/1, Sigmoid_brake/1(Change_time)  "Time"
  Brake_Switch/1 -> Abs2/1  "Brake"
  Clock1/1 -> Switch3/1
  Switch4/1 -> Switch4/3, Sigmoid_brake/2(Old brake)  "Old brake"
  Delay3/1 -> Switch4/1
  Sigmoid_brake/1(brake_out) -> Delay3/1, Scope/2, Brake_Switch2/3  "Smoothed Brake"
  Square1/1 -> Sum/1
  Constant1/1 -> Sum/2
  Sum/1 -> Sqrt1/1
  Divide2/1 -> Divide/1
  Sqrt1/1 -> Divide/2
  Gain4/1 -> Abs4/1
  Divide/1 -> Add/3
  Add/1 -> Saturation/1
  Saturation/1 -> Scope3/1, Throttle_Switch/1  "Throttle"
  Square2/1 -> Sum1/1
  Gain6/1 -> Abs5/1
  Divide1/1 -> Add1/3
  Constant2/1 -> Sum1/2
  Divide3/1 -> Divide1/1
  Sum1/1 -> Sqrt2/1
  Add1/1 -> Saturation1/1
  Sqrt2/1 -> Divide1/2
  Grade/1 -> Gain1/1, Divide2/1, Square1/1, Gain/1, Divide3/1, Square2/1
  Saturation1/1 -> Brake_Switch/3  "Brake"
  Constant4/1 -> Divide3/2, Divide2/2
  Divide4/1 -> Add1/1
  Gain/1 -> Abs/1
  Abs/1 -> Divide4/2
  Abs1/1 -> Divide5/2
  Gain1/1 -> Abs1/1
  Divide5/1 -> Add/1
  P/1 -> Divide4/1, Divide5/1
  Delay/1 -> Equal/1
  Constant/1 -> NotEqual/1, Equal/2
  Equal/1 -> AND/1, Scope2/2  "EqualZero"
  NotEqual/1 -> Scope2/3, AND/2  "NEqualZero"
  OR/1 -> Switch1/2, Switch2/2
  AND/1 -> Scope2/4, OR/1  "Both"
  Abs2/1 -> Scope/3, Sigmoid_brake/3(New brake)
  Abs3/1 -> Scope2/1, Delay/1, NotEqual/2, Scope1/2, Sigmoid_throttle/3(New thr)
  Abs4/1 -> Add/2
  Abs5/1 -> Add1/2

== system CCModel_61/Cruise Control/Version 6.3/Apply_Grade ==
  note: This has not been implemented but may be helpful
  note: +(2/5)|P|
  note: x is u, which is linear and g is grade which is sigmoided
  U_in : Inport
  Grade : Inport  Port=2
  Add : Sum
  Add Constant : Bias  Bias=1  SaturateOnIntegerOverflow=off
  Divide : Product  Inputs=*/
  Gain : Gain  Gain=0.8
  Gain1 : Gain  Gain=0.25
  Scope : Scope  NumInputPorts=2
  Sqrt : Sqrt
  Square : Math  Operator=square
  U_Out : Outport
  wires:
  U_in/1 -> Scope/1, Gain/1
  Square/1 -> Add Constant/1
  Add Constant/1 -> Sqrt/1
  Grade/1 -> Gain1/1, Square/1
  Gain1/1 -> Divide/1
  Sqrt/1 -> Divide/2
  Divide/1 -> Add/2
  Gain/1 -> Add/1
  Add/1 -> Scope/2, U_Out/1

== system CCModel_61/Cruise Control/Version 6.3/Detect Change ==
  note: This subsystem detects either a change in the reference velocity, or the driver releasing one of the pedals. It outputs the time of the change, the value of u just before the change, and a boolean "hasChanged" value
  desired_velocity : Inport
  throttle_const : Inport  Port=2
  brake_const : Inport  Port=3
  Smoothed u : Inport  Port=4
  (False) : Constant  Value=0
  (True) : Constant
  AND : Logic  IconShape=distinctive  AllPortsSameDT=off  OutDataTypeStr=boolean
  Clock : Clock
  Constant : Constant  Value=0.01
  Delay : Delay  DelayLength=1
  Delay1 : Delay  DelayLength=1
  Detect Change : simulink/Logic and Bit Operations/Detect Change  vinit=0  OutDataTypeStr=boolean
  Detect Change1 : simulink/Logic and Bit Operations/Detect Change  vinit=0  OutDataTypeStr=boolean
  Max : MinMax  Function=max  Inputs=2
  Max1 : MinMax  Function=max  Inputs=2
  OR : Logic  Operator=OR  IconShape=distinctive  AllPortsSameDT=off  OutDataTypeStr=boolean
  Pedal_threshold : Constant
  Scope : Scope
  Subtract : Sum  Inputs=+-
  Switch : Switch  Criteria=u2 > Threshold  SaturateOnIntegerOverflow=off  InputSameDT=off
  Switch1 : Switch  Criteria=u2 > Threshold  SaturateOnIntegerOverflow=off  InputSameDT=off
  Switch2 : Switch  Criteria=u2 > Threshold  SaturateOnIntegerOverflow=off  InputSameDT=off
  Change_time : Outport
  Old u : Outport  Port=2
  hasChanged : Outport  Port=3
  wires:
  desired_velocity/1 -> Detect Change/1
  Detect Change/1 -> OR/1
  OR/1 -> Switch/2, Switch2/2, hasChanged/1
  Switch1/1 -> Detect Change1/1, Delay1/1
  AND/1 -> OR/2
  Clock/1 -> Switch/1
  Max/1 -> Subtract/1
  (True)/1 -> Switch1/1
  brake_const/1 -> Max/2
  Pedal_threshold/1 -> Subtract/2
  Subtract/1 -> Switch1/2
  (False)/1 -> Switch1/3
  throttle_const/1 -> Max/1
  Switch2/1 -> Switch2/3, Max1/1
  Delay/1 -> Switch2/1
  Switch/1 -> Switch/3, Scope/1, Change_time/1
  Smoothed u/1 -> Delay/1
  Detect Change1/1 -> AND/2
  Delay1/1 -> AND/1
  Constant/1 -> Max1/2
  Max1/1 -> Old u/1

== system CCModel_61/Cruise Control/Version 6.3/PID Controller ==
  note: Typical PID controller, outputs a value between -100 and 100
  error : Inport
  Grade : Inport  Port=2
  Add : Sum
  Add1 : Sum
  Derivative : Derivative
  GKi : Gain  Gain=0
  GKp : Gain  Gain=0
  Integrator : Integrator
  Integrator1 : Integrator
  Kd : Gain  Gain=0.1
  Ki : Gain  Gain=0.03
  Kp : Gain  Gain=3
  Saturation : Saturate  UpperLimit=100  LowerLimit=-100
  Scope1 : Scope  NumInputPorts=3
  Sum : Sum  Inputs=+++
  u : Outport
  wires:
  Integrator/1 -> Ki/1
  error/1 -> Integrator/1, Kp/1, Derivative/1  "D"
  Kp/1 -> Scope1/1, Sum/2  "P"
  Ki/1 -> Sum/1, Scope1/2  "I"
  Saturation/1 -> u/1
  Derivative/1 -> Kd/1
  Kd/1 -> Scope1/3, Sum/3  "D"
  Sum/1 -> Add1/1
  Add1/1 -> Saturation/1
  Grade/1 -> Integrator1/1, GKp/1
  Integrator1/1 -> GKi/1
  GKi/1 -> Add/1
  GKp/1 -> Add/2
  Add/1 -> Add1/2

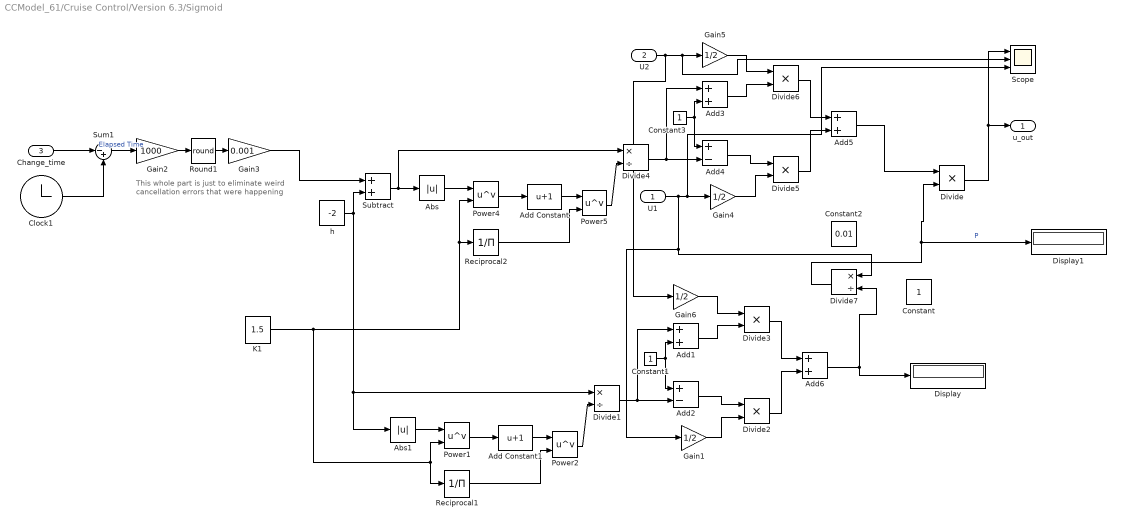
== system CCModel_61/Cruise Control/Version 6.3/Sigmoid ==
  note: This whole part is just to eliminate weird cancellation errors that were happening
  U1 : Inport
  U2 : Inport  Port=2
  Change_time : Inport  Port=3
  Abs : Abs  SaturateOnIntegerOverflow=off
  Abs1 : Abs  SaturateOnIntegerOverflow=off
  Add Constant : Bias  Bias=1  SaturateOnIntegerOverflow=off
  Add Constant1 : Bias  Bias=1  SaturateOnIntegerOverflow=off
  Add{1,3,5..6} (4 alike) : Sum
  Add2 : Sum  Inputs=+-
  Add4 : Sum  Inputs=+-
  Clock1 : Clock
  Constant : Constant
  Constant1 : Constant
  Constant2 : Constant  Value=0.01
  Constant3 : Constant
  Display : Display
  Display1 : Display
  Divide{,2..3,5..6} (5 alike) : Product  Inputs=**
  Divide1 : Product  Inputs=*/
  Divide4 : Product  Inputs=*/
  Divide7 : Product  Inputs=*/
  Gain{1,4..6} (4 alike) : Gain  Gain=1/2
  Gain2 : Gain  Gain=1000
  Gain3 : Gain  Gain=0.001
  K1 : Constant  Value=1.5
  Power{1..2,4..5} (4 alike) : Math  Operator=pow
  Reciprocal1 : Product  Inputs=/
  Reciprocal2 : Product  Inputs=/
  Round1 : Rounding  Operator=round
  Scope : Scope  NumInputPorts=3
  Subtract : Sum
  Sum1 : Sum  Inputs=|-+
  h : Constant  Value=-2
  u_out : Outport
  wires:
  Gain6/1 -> Divide3/1
  Divide2/1 -> Add6/2
  Divide3/1 -> Add6/1
  Gain1/1 -> Divide2/2
  Divide1/1 -> Add1/1, Add2/2
  Add2/1 -> Divide2/1
  Add1/1 -> Divide3/2
  Constant1/1 -> Add1/2, Add2/1
  Power1/1 -> Add Constant1/1
  Add5/1 -> Divide/1
  h/1 -> Divide1/1, Abs1/1, Subtract/2
  Add3/1 -> Divide6/2
  Add4/1 -> Divide5/1
  Constant3/1 -> Add3/2, Add4/1
  Divide/1 -> Scope/1, u_out/1
  Power5/1 -> Divide4/2
  Reciprocal2/1 -> Power5/2
  K1/1 -> Power1/2, Reciprocal1/1, Power4/2, Reciprocal2/1
  Abs1/1 -> Power1/1
  Gain5/1 -> Divide6/1
  Change_time/1 -> Sum1/1
  Abs/1 -> Power4/1
  Divide5/1 -> Add5/2
  Add6/1 -> Display/1, Divide7/2
  Clock1/1 -> Sum1/2
  Gain4/1 -> Divide5/2
  Gain3/1 -> Subtract/1
  U2/1 -> Gain6/1, Scope/2, Gain5/1
  Power2/1 -> Divide1/2
  Round1/1 -> Gain3/1
  Power4/1 -> Add Constant/1
  Add Constant1/1 -> Power2/1
  Gain2/1 -> Round1/1
  Add Constant/1 -> Power5/1
  Subtract/1 -> Divide4/1, Abs/1
  U1/1 -> Divide7/1, Gain1/1, Scope/3, Gain4/1
  Divide6/1 -> Add5/1
  Sum1/1 -> Gain2/1  "Elapsed Time"
  Divide4/1 -> Add3/1, Add4/2
  Reciprocal1/1 -> Power2/2
  Divide7/1 -> Divide/2, Display1/1  "P"

== system CCModel_61/Cruise Control/Version 6.3/Switches ==
  note: Apply sigmoid curving to the throttle and brake
  U : Inport
  Throttle_In : Inport  Port=2
  Brake_In : Inport  Port=3
  Brake_Switch : Switch  Criteria=u2 > Threshold  SaturateOnIntegerOverflow=off  InputSameDT=off
  Brake_Switch2 : Switch  Criteria=u2 > Threshold  Threshold=5  SaturateOnIntegerOverflow=off  InputSameDT=off
  Constant1 : Constant  Value=10
  Constant2 : Constant  Value=10
  Exp : Math
  Exp1 : Math
  Gain : Gain  Gain=1/10
  Gain1 : Gain  Gain=0.9
  Gain2 : Gain  Gain=10
  Gain3 : Gain  Gain=1/10
  Gain4 : Gain  Gain=0.9
  Gain5 : Gain  Gain=10
  Gain6 : Gain  Gain=-1
  Max : MinMax  Function=max  Inputs=2
  Plus : Sum
  Plus1 : Sum
  Ramp : simulink/Sources/Ramp  slope=1  start=0  InitialOutput=-100
  Saturation2 : Saturate  UpperLimit=100  LowerLimit=-100
  Scope4 : Scope  NumInputPorts=3
  Throttle_Switch : Switch  Criteria=u2 > Threshold  SaturateOnIntegerOverflow=off  InputSameDT=off
  Throttle_Switch2 : Switch  Criteria=u2 > Threshold  Threshold=5  SaturateOnIntegerOverflow=off  InputSameDT=off
  Throttle : Outport
  Brake : Outport  Port=2
  wires:
  Saturation2/1 -> Gain1/1, Throttle_Switch/2, Scope4/1, Gain6/1
  Throttle_Switch/1 -> Throttle_Switch2/3  "Throttle"
  Gain1/1 -> Gain/1, Plus/1
  Constant1/1 -> Plus/2
  Plus/1 -> Throttle_Switch/1
  Gain/1 -> Exp/1
  Exp/1 -> Gain2/1
  Gain2/1 -> Throttle_Switch/3
  Gain5/1 -> Brake_Switch/3
  Constant2/1 -> Plus1/2
  Gain3/1 -> Exp1/1
  Gain4/1 -> Gain3/1, Plus1/1
  Plus1/1 -> Brake_Switch/1
  Exp1/1 -> Gain5/1
  Gain6/1 -> Gain4/1, Brake_Switch/2
  Max/1 -> Throttle_Switch2/2, Brake_Switch2/2
  Throttle_In/1 -> Throttle_Switch2/1, Max/1
  Brake_In/1 -> Brake_Switch2/1, Max/2
  Brake_Switch/1 -> Brake_Switch2/3  "Brake"
  Brake_Switch2/1 -> Scope4/3, Brake/1
  Throttle_Switch2/1 -> Scope4/2, Throttle/1
  U/1 -> Saturation2/1

== system CCModel_61/Cruise Control/Version 6.4/Apply_Grade ==
  note: This has not been implemented but may be helpful
  note: +(2/5)|P|
  note: x is u, which is linear and g is grade which is sigmoided
  U_in : Inport
  Grade : Inport  Port=2
  Add : Sum
  Add Constant : Bias  Bias=1  SaturateOnIntegerOverflow=off
  Divide : Product  Inputs=*/
  Gain : Gain  Gain=0.8
  Gain1 : Gain  Gain=0.25
  Scope : Scope  NumInputPorts=2
  Sqrt : Sqrt
  Square : Math  Operator=square
  U_Out : Outport
  wires:
  U_in/1 -> Scope/1, Gain/1
  Square/1 -> Add Constant/1
  Add Constant/1 -> Sqrt/1
  Grade/1 -> Gain1/1, Square/1
  Gain1/1 -> Divide/1
  Sqrt/1 -> Divide/2
  Divide/1 -> Add/2
  Gain/1 -> Add/1
  Add/1 -> Scope/2, U_Out/1

== system CCModel_61/Cruise Control/Version 6.4/Detect Change ==
  note: This subsystem detects either a change in the reference velocity, or the driver releasing one of the pedals. It outputs the time of the change, the value of u just before the change, and a boolean "hasChanged" value
  desired_velocity : Inport
  throttle_const : Inport  Port=2
  brake_const : Inport  Port=3
  Smoothed u : Inport  Port=4
  (False) : Constant  Value=0
  (True) : Constant
  AND : Logic  IconShape=distinctive  AllPortsSameDT=off  OutDataTypeStr=boolean
  Clock : Clock
  Constant : Constant  Value=0.01
  Delay : Delay  DelayLength=1
  Delay1 : Delay  DelayLength=1
  Detect Change : simulink/Logic and Bit Operations/Detect Change  vinit=0  OutDataTypeStr=boolean
  Detect Change1 : simulink/Logic and Bit Operations/Detect Change  vinit=0  OutDataTypeStr=boolean
  Max : MinMax  Function=max  Inputs=2
  Max1 : MinMax  Function=max  Inputs=2
  OR : Logic  Operator=OR  IconShape=distinctive  AllPortsSameDT=off  OutDataTypeStr=boolean
  Pedal_threshold : Constant
  Scope : Scope
  Subtract : Sum  Inputs=+-
  Switch : Switch  Criteria=u2 > Threshold  SaturateOnIntegerOverflow=off  InputSameDT=off
  Switch1 : Switch  Criteria=u2 > Threshold  SaturateOnIntegerOverflow=off  InputSameDT=off
  Switch2 : Switch  Criteria=u2 > Threshold  SaturateOnIntegerOverflow=off  InputSameDT=off
  Change_time : Outport
  Old u : Outport  Port=2
  hasChanged : Outport  Port=3
  wires:
  desired_velocity/1 -> Detect Change/1
  Detect Change/1 -> OR/1
  OR/1 -> Switch/2, Switch2/2, hasChanged/1
  Switch1/1 -> Detect Change1/1, Delay1/1
  AND/1 -> OR/2
  Clock/1 -> Switch/1
  Max/1 -> Subtract/1
  (True)/1 -> Switch1/1
  brake_const/1 -> Max/2
  Pedal_threshold/1 -> Subtract/2
  Subtract/1 -> Switch1/2
  (False)/1 -> Switch1/3
  throttle_const/1 -> Max/1
  Switch2/1 -> Switch2/3, Max1/1
  Delay/1 -> Switch2/1
  Switch/1 -> Switch/3, Scope/1, Change_time/1
  Smoothed u/1 -> Delay/1
  Detect Change1/1 -> AND/2
  Delay1/1 -> AND/1
  Constant/1 -> Max1/2
  Max1/1 -> Old u/1

== system CCModel_61/Cruise Control/Version 6.4/PID Controller ==
  note: Typical PID controller, outputs a value between -100 and 100
  error : Inport
  Grade : Inport  Port=2
  Add : Sum
  Add1 : Sum
  Derivative : Derivative
  GKi : Gain  Gain=0
  GKp : Gain  Gain=0
  Integrator : Integrator
  Integrator1 : Integrator
  Kd : Gain  Gain=0.1
  Ki : Gain  Gain=0.03
  Kp : Gain  Gain=3
  Saturation : Saturate  UpperLimit=100  LowerLimit=-100
  Scope1 : Scope  NumInputPorts=3
  Sum : Sum  Inputs=+++
  u : Outport
  wires:
  Integrator/1 -> Ki/1
  error/1 -> Integrator/1, Kp/1, Derivative/1  "D"
  Kp/1 -> Scope1/1, Sum/2  "P"
  Ki/1 -> Sum/1, Scope1/2  "I"
  Saturation/1 -> u/1
  Derivative/1 -> Kd/1
  Kd/1 -> Scope1/3, Sum/3  "D"
  Sum/1 -> Add1/1
  Add1/1 -> Saturation/1
  Grade/1 -> Integrator1/1, GKp/1
  Integrator1/1 -> GKi/1
  GKi/1 -> Add/1
  GKp/1 -> Add/2
  Add/1 -> Add1/2
